simulink model "cantx_0x191"  (R2015a)
settings: Solver=ode45  SolverMode=SingleTasking  StartTime=0.0  StopTime=10.0  RelTol=1e-3
libraries: simulink x6
settings Model: CovMetricSettings=dwe  CovHtmlReporting=off  covSaveCumulativeToWorkspaceVar=off  CovSaveSingleToWorkspaceVar=off  CovExternalEMLEnable=on  Creator=Castiel  LastModifiedBy=Castiel
settings DataIOCC: LimitDataPoints=off  SaveFormat=Dataset  ReturnWorkspaceOutputs=on
settings DebuggingCC: UnconnectedInputMsg=none  UnconnectedOutputMsg=none  UnconnectedLineMsg=none  SFUnexpectedBacktrackingDiag=error  SFNoUnconditionalDefaultTransitionDiag=error
settings HardwareCC: ProdBitPerPointer=64  ProdLargestAtomicFloat=Float  ProdIntDivRoundTo=Zero  ProdEndianess=LittleEndian  ProdHWDeviceType=Specified
settings ModelReferenceCC: PropagateSignalLabelsOutOfModel=on
settings SFSimCC: SimUseLocalCustomCode=on
settings RTWCC: RTWUseLocalCustomCode=on
settings GRTTargetCC: TargetLangStandard=C99 (ISO)

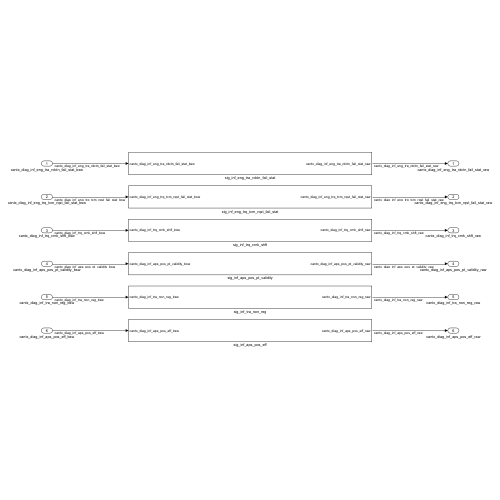
[thumbnail: Simulink's stored preview of the top-level diagram]
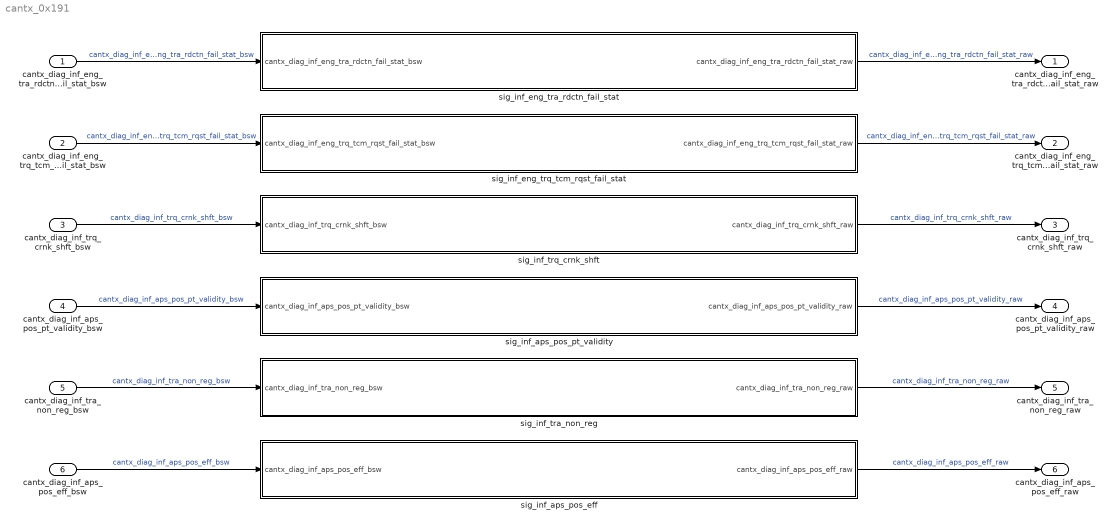
== system cantx_0x191 ==
  cantx_diag_inf_eng_tra_rdctn_fail_stat_bsw : Inport
  cantx_diag_inf_eng_trq_tcm_rqst_fail_stat_bsw : Inport  Port=2
  cantx_diag_inf_trq_crnk_shft_bsw : Inport  Port=3
  cantx_diag_inf_aps_pos_pt_validity_bsw : Inport  Port=4
  cantx_diag_inf_tra_non_reg_bsw : Inport  Port=5
  cantx_diag_inf_aps_pos_eff_bsw : Inport  Port=6
  sig_inf_aps_pos_eff : Subsystem
  sig_inf_aps_pos_pt_validity : Subsystem
  sig_inf_eng_tra_rdctn_fail_stat : Subsystem
  sig_inf_eng_trq_tcm_rqst_fail_stat : Subsystem
  sig_inf_tra_non_reg : Subsystem
  sig_inf_trq_crnk_shft : Subsystem
  cantx_diag_inf_eng_tra_rdctn_fail_stat_raw : Outport
  cantx_diag_inf_eng_trq_tcm_rqst_fail_stat_raw : Outport  Port=2
  cantx_diag_inf_trq_crnk_shft_raw : Outport  Port=3
  cantx_diag_inf_aps_pos_pt_validity_raw : Outport  Port=4
  cantx_diag_inf_tra_non_reg_raw : Outport  Port=5
  cantx_diag_inf_aps_pos_eff_raw : Outport  Port=6
  wires:
  cantx_diag_inf_eng_tra_rdctn_fail_stat_bsw/1 -> sig_inf_eng_tra_rdctn_fail_stat/1(cantx_diag_inf_eng_tra_rdctn_fail_stat_bsw)  "cantx_diag_inf_eng_tra_rdctn_fail_stat_bsw"
  sig_inf_eng_tra_rdctn_fail_stat/1(cantx_diag_inf_eng_tra_rdctn_fail_stat_raw) -> cantx_diag_inf_eng_tra_rdctn_fail_stat_raw/1  "cantx_diag_inf_eng_tra_rdctn_fail_stat_raw"
  cantx_diag_inf_eng_trq_tcm_rqst_fail_stat_bsw/1 -> sig_inf_eng_trq_tcm_rqst_fail_stat/1(cantx_diag_inf_eng_trq_tcm_rqst_fail_stat_bsw)  "cantx_diag_inf_eng_trq_tcm_rqst_fail_stat_bsw"
  sig_inf_eng_trq_tcm_rqst_fail_stat/1(cantx_diag_inf_eng_trq_tcm_rqst_fail_stat_raw) -> cantx_diag_inf_eng_trq_tcm_rqst_fail_stat_raw/1  "cantx_diag_inf_eng_trq_tcm_rqst_fail_stat_raw"
  cantx_diag_inf_trq_crnk_shft_bsw/1 -> sig_inf_trq_crnk_shft/1(cantx_diag_inf_trq_crnk_shft_bsw)  "cantx_diag_inf_trq_crnk_shft_bsw"
  sig_inf_trq_crnk_shft/1(cantx_diag_inf_trq_crnk_shft_raw) -> cantx_diag_inf_trq_crnk_shft_raw/1  "cantx_diag_inf_trq_crnk_shft_raw"
  cantx_diag_inf_aps_pos_pt_validity_bsw/1 -> sig_inf_aps_pos_pt_validity/1(cantx_diag_inf_aps_pos_pt_validity_bsw)  "cantx_diag_inf_aps_pos_pt_validity_bsw"
  sig_inf_aps_pos_pt_validity/1(cantx_diag_inf_aps_pos_pt_validity_raw) -> cantx_diag_inf_aps_pos_pt_validity_raw/1  "cantx_diag_inf_aps_pos_pt_validity_raw"
  cantx_diag_inf_tra_non_reg_bsw/1 -> sig_inf_tra_non_reg/1(cantx_diag_inf_tra_non_reg_bsw)  "cantx_diag_inf_tra_non_reg_bsw"
  sig_inf_tra_non_reg/1(cantx_diag_inf_tra_non_reg_raw) -> cantx_diag_inf_tra_non_reg_raw/1  "cantx_diag_inf_tra_non_reg_raw"
  cantx_diag_inf_aps_pos_eff_bsw/1 -> sig_inf_aps_pos_eff/1(cantx_diag_inf_aps_pos_eff_bsw)  "cantx_diag_inf_aps_pos_eff_bsw"
  sig_inf_aps_pos_eff/1(cantx_diag_inf_aps_pos_eff_raw) -> cantx_diag_inf_aps_pos_eff_raw/1  "cantx_diag_inf_aps_pos_eff_raw"

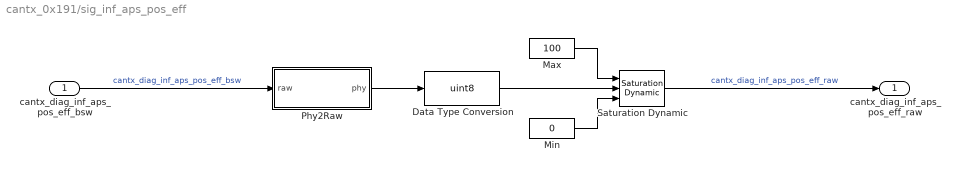
== system cantx_0x191/sig_inf_aps_pos_eff ==
  cantx_diag_inf_aps_pos_eff_bsw : Inport
  Data Type Conversion : DataTypeConversion  OutDataTypeStr=uint8
  Max : Constant  Value=100
  Min : Constant  Value=0
  Phy2Raw : Subsystem  mask{Offset=0, Factor=100/255}
      mask Callback Offset:
      | offset = get_param(gcb, 'Offset');
      |     set_param([gcb, '/Offset'], 'Value', offset);
      mask Callback Factor:
      | factor = get_param(gcb, 'Factor');
      |     set_param([gcb, '/Factor'], 'Value', factor);
      mask Display:
      | disp(['Offset = ', get_param(gcb, 'Offset'), '\n\n']);
      | disp(['Factor = ', get_param(gcb, 'Factor')]);
  Saturation Dynamic : simulink/Discontinuities/Saturation Dynamic  OutMin=[]  OutMax=[]  OutDataTypeStr=Inherit: Same as second input  OutDataType=fixdt(1, 16)  OutScaling=2^-10  DoSatur=off
  cantx_diag_inf_aps_pos_eff_raw : Outport
  wires:
  Saturation Dynamic/1 -> cantx_diag_inf_aps_pos_eff_raw/1  "cantx_diag_inf_aps_pos_eff_raw"
  Phy2Raw/1(phy) -> Data Type Conversion/1
  Data Type Conversion/1 -> Saturation Dynamic/2
  cantx_diag_inf_aps_pos_eff_bsw/1 -> Phy2Raw/1(raw)  "cantx_diag_inf_aps_pos_eff_bsw"
  Min/1 -> Saturation Dynamic/3
  Max/1 -> Saturation Dynamic/1

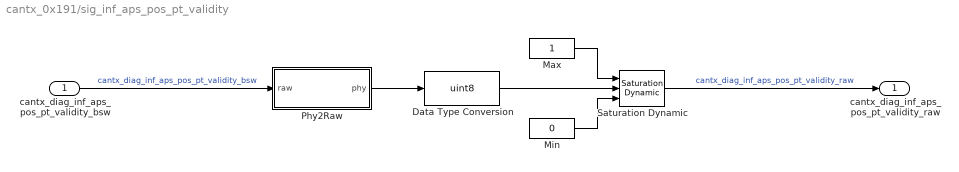
== system cantx_0x191/sig_inf_aps_pos_pt_validity ==
  cantx_diag_inf_aps_pos_pt_validity_bsw : Inport
  Data Type Conversion : DataTypeConversion  OutDataTypeStr=uint8
  Max : Constant
  Min : Constant  Value=0
  Phy2Raw : Subsystem  mask{Offset=0, Factor=1}
      mask Callback Offset:
      | offset = get_param(gcb, 'Offset');
      |     set_param([gcb, '/Offset'], 'Value', offset);
      mask Callback Factor:
      | factor = get_param(gcb, 'Factor');
      |     set_param([gcb, '/Factor'], 'Value', factor);
      mask Display:
      | disp(['Offset = ', get_param(gcb, 'Offset'), '\n\n']);
      | disp(['Factor = ', get_param(gcb, 'Factor')]);
  Saturation Dynamic : simulink/Discontinuities/Saturation Dynamic  OutMin=[]  OutMax=[]  OutDataTypeStr=Inherit: Same as second input  OutDataType=fixdt(1, 16)  OutScaling=2^-10  DoSatur=off
  cantx_diag_inf_aps_pos_pt_validity_raw : Outport
  wires:
  Saturation Dynamic/1 -> cantx_diag_inf_aps_pos_pt_validity_raw/1  "cantx_diag_inf_aps_pos_pt_validity_raw"
  Phy2Raw/1(phy) -> Data Type Conversion/1
  Data Type Conversion/1 -> Saturation Dynamic/2
  cantx_diag_inf_aps_pos_pt_validity_bsw/1 -> Phy2Raw/1(raw)  "cantx_diag_inf_aps_pos_pt_validity_bsw"
  Min/1 -> Saturation Dynamic/3
  Max/1 -> Saturation Dynamic/1

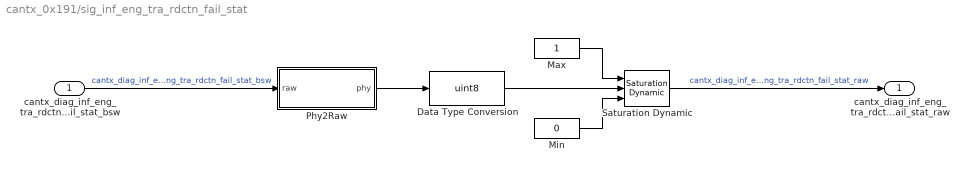
== system cantx_0x191/sig_inf_eng_tra_rdctn_fail_stat ==
  cantx_diag_inf_eng_tra_rdctn_fail_stat_bsw : Inport
  Data Type Conversion : DataTypeConversion  OutDataTypeStr=uint8
  Max : Constant
  Min : Constant  Value=0
  Phy2Raw : Subsystem  mask{Offset=0, Factor=1}
      mask Callback Offset:
      | offset = get_param(gcb, 'Offset');
      |     set_param([gcb, '/Offset'], 'Value', offset);
      mask Callback Factor:
      | factor = get_param(gcb, 'Factor');
      |     set_param([gcb, '/Factor'], 'Value', factor);
      mask Display:
      | disp(['Offset = ', get_param(gcb, 'Offset'), '\n\n']);
      | disp(['Factor = ', get_param(gcb, 'Factor')]);
  Saturation Dynamic : simulink/Discontinuities/Saturation Dynamic  OutMin=[]  OutMax=[]  OutDataTypeStr=Inherit: Same as second input  OutDataType=fixdt(1, 16)  OutScaling=2^-10  DoSatur=off
  cantx_diag_inf_eng_tra_rdctn_fail_stat_raw : Outport
  wires:
  Saturation Dynamic/1 -> cantx_diag_inf_eng_tra_rdctn_fail_stat_raw/1  "cantx_diag_inf_eng_tra_rdctn_fail_stat_raw"
  Phy2Raw/1(phy) -> Data Type Conversion/1
  Data Type Conversion/1 -> Saturation Dynamic/2
  cantx_diag_inf_eng_tra_rdctn_fail_stat_bsw/1 -> Phy2Raw/1(raw)  "cantx_diag_inf_eng_tra_rdctn_fail_stat_bsw"
  Min/1 -> Saturation Dynamic/3
  Max/1 -> Saturation Dynamic/1

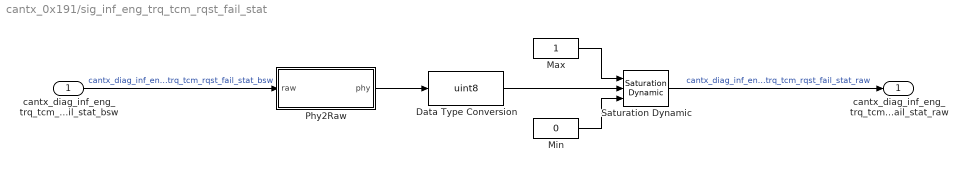
== system cantx_0x191/sig_inf_eng_trq_tcm_rqst_fail_stat ==
  cantx_diag_inf_eng_trq_tcm_rqst_fail_stat_bsw : Inport
  Data Type Conversion : DataTypeConversion  OutDataTypeStr=uint8
  Max : Constant
  Min : Constant  Value=0
  Phy2Raw : Subsystem  mask{Offset=0, Factor=1}
      mask Callback Offset:
      | offset = get_param(gcb, 'Offset');
      |     set_param([gcb, '/Offset'], 'Value', offset);
      mask Callback Factor:
      | factor = get_param(gcb, 'Factor');
      |     set_param([gcb, '/Factor'], 'Value', factor);
      mask Display:
      | disp(['Offset = ', get_param(gcb, 'Offset'), '\n\n']);
      | disp(['Factor = ', get_param(gcb, 'Factor')]);
  Saturation Dynamic : simulink/Discontinuities/Saturation Dynamic  OutMin=[]  OutMax=[]  OutDataTypeStr=Inherit: Same as second input  OutDataType=fixdt(1, 16)  OutScaling=2^-10  DoSatur=off
  cantx_diag_inf_eng_trq_tcm_rqst_fail_stat_raw : Outport
  wires:
  Saturation Dynamic/1 -> cantx_diag_inf_eng_trq_tcm_rqst_fail_stat_raw/1  "cantx_diag_inf_eng_trq_tcm_rqst_fail_stat_raw"
  Phy2Raw/1(phy) -> Data Type Conversion/1
  Data Type Conversion/1 -> Saturation Dynamic/2
  cantx_diag_inf_eng_trq_tcm_rqst_fail_stat_bsw/1 -> Phy2Raw/1(raw)  "cantx_diag_inf_eng_trq_tcm_rqst_fail_stat_bsw"
  Min/1 -> Saturation Dynamic/3
  Max/1 -> Saturation Dynamic/1

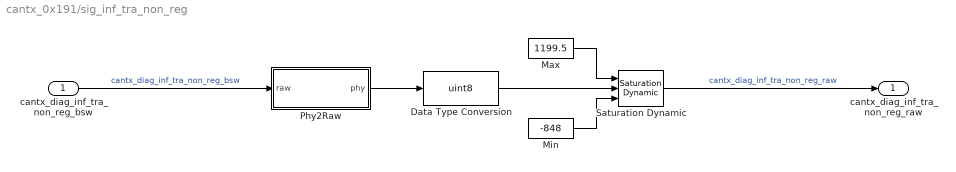
== system cantx_0x191/sig_inf_tra_non_reg ==
  cantx_diag_inf_tra_non_reg_bsw : Inport
  Data Type Conversion : DataTypeConversion  OutDataTypeStr=uint8
  Max : Constant  Value=1199.5
  Min : Constant  Value=-848
  Phy2Raw : Subsystem  mask{Offset=-848, Factor=0.5}
      mask Callback Offset:
      | offset = get_param(gcb, 'Offset');
      |     set_param([gcb, '/Offset'], 'Value', offset);
      mask Callback Factor:
      | factor = get_param(gcb, 'Factor');
      |     set_param([gcb, '/Factor'], 'Value', factor);
      mask Display:
      | disp(['Offset = ', get_param(gcb, 'Offset'), '\n\n']);
      | disp(['Factor = ', get_param(gcb, 'Factor')]);
  Saturation Dynamic : simulink/Discontinuities/Saturation Dynamic  OutMin=[]  OutMax=[]  OutDataTypeStr=Inherit: Same as second input  OutDataType=fixdt(1, 16)  OutScaling=2^-10  DoSatur=off
  cantx_diag_inf_tra_non_reg_raw : Outport
  wires:
  Saturation Dynamic/1 -> cantx_diag_inf_tra_non_reg_raw/1  "cantx_diag_inf_tra_non_reg_raw"
  Phy2Raw/1(phy) -> Data Type Conversion/1
  Data Type Conversion/1 -> Saturation Dynamic/2
  cantx_diag_inf_tra_non_reg_bsw/1 -> Phy2Raw/1(raw)  "cantx_diag_inf_tra_non_reg_bsw"
  Min/1 -> Saturation Dynamic/3
  Max/1 -> Saturation Dynamic/1

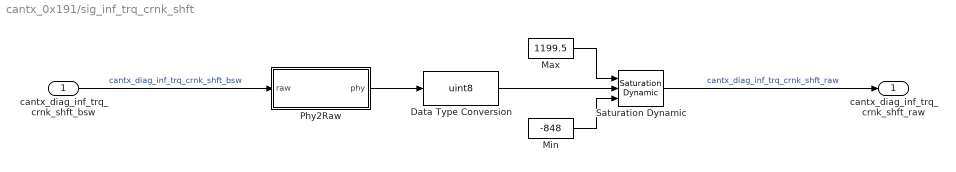
== system cantx_0x191/sig_inf_trq_crnk_shft ==
  cantx_diag_inf_trq_crnk_shft_bsw : Inport
  Data Type Conversion : DataTypeConversion  OutDataTypeStr=uint8
  Max : Constant  Value=1199.5
  Min : Constant  Value=-848
  Phy2Raw : Subsystem  mask{Offset=-848, Factor=0.5}
      mask Callback Offset:
      | offset = get_param(gcb, 'Offset');
      |     set_param([gcb, '/Offset'], 'Value', offset);
      mask Callback Factor:
      | factor = get_param(gcb, 'Factor');
      |     set_param([gcb, '/Factor'], 'Value', factor);
      mask Display:
      | disp(['Offset = ', get_param(gcb, 'Offset'), '\n\n']);
      | disp(['Factor = ', get_param(gcb, 'Factor')]);
  Saturation Dynamic : simulink/Discontinuities/Saturation Dynamic  OutMin=[]  OutMax=[]  OutDataTypeStr=Inherit: Same as second input  OutDataType=fixdt(1, 16)  OutScaling=2^-10  DoSatur=off
  cantx_diag_inf_trq_crnk_shft_raw : Outport
  wires:
  Saturation Dynamic/1 -> cantx_diag_inf_trq_crnk_shft_raw/1  "cantx_diag_inf_trq_crnk_shft_raw"
  Phy2Raw/1(phy) -> Data Type Conversion/1
  Data Type Conversion/1 -> Saturation Dynamic/2
  cantx_diag_inf_trq_crnk_shft_bsw/1 -> Phy2Raw/1(raw)  "cantx_diag_inf_trq_crnk_shft_bsw"
  Min/1 -> Saturation Dynamic/3
  Max/1 -> Saturation Dynamic/1

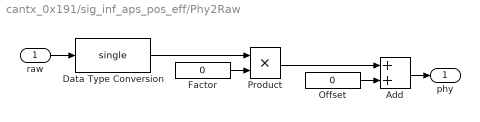
== system cantx_0x191/sig_inf_aps_pos_eff/Phy2Raw ==
  raw : Inport
  Add : Sum
  Data Type Conversion : DataTypeConversion  OutDataTypeStr=single
  Factor : Constant  Value=0
  Offset : Constant  Value=0
  Product : Product
  phy : Outport
  wires:
  Add/1 -> phy/1
  Factor/1 -> Product/2
  Data Type Conversion/1 -> Product/1
  Offset/1 -> Add/2
  Product/1 -> Add/1
  raw/1 -> Data Type Conversion/1

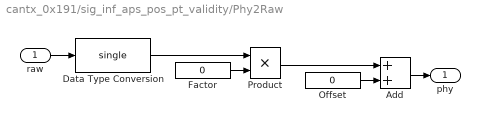
== system cantx_0x191/sig_inf_aps_pos_pt_validity/Phy2Raw ==
  raw : Inport
  Add : Sum
  Data Type Conversion : DataTypeConversion  OutDataTypeStr=single
  Factor : Constant  Value=0
  Offset : Constant  Value=0
  Product : Product
  phy : Outport
  wires:
  Add/1 -> phy/1
  Factor/1 -> Product/2
  Data Type Conversion/1 -> Product/1
  Offset/1 -> Add/2
  Product/1 -> Add/1
  raw/1 -> Data Type Conversion/1

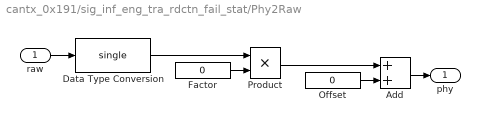
== system cantx_0x191/sig_inf_eng_tra_rdctn_fail_stat/Phy2Raw ==
  raw : Inport
  Add : Sum
  Data Type Conversion : DataTypeConversion  OutDataTypeStr=single
  Factor : Constant  Value=0
  Offset : Constant  Value=0
  Product : Product
  phy : Outport
  wires:
  Add/1 -> phy/1
  Factor/1 -> Product/2
  Data Type Conversion/1 -> Product/1
  Offset/1 -> Add/2
  Product/1 -> Add/1
  raw/1 -> Data Type Conversion/1

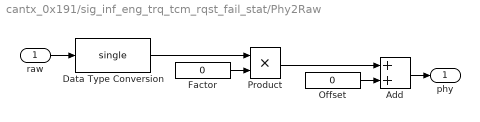
== system cantx_0x191/sig_inf_eng_trq_tcm_rqst_fail_stat/Phy2Raw ==
  raw : Inport
  Add : Sum
  Data Type Conversion : DataTypeConversion  OutDataTypeStr=single
  Factor : Constant  Value=0
  Offset : Constant  Value=0
  Product : Product
  phy : Outport
  wires:
  Add/1 -> phy/1
  Factor/1 -> Product/2
  Data Type Conversion/1 -> Product/1
  Offset/1 -> Add/2
  Product/1 -> Add/1
  raw/1 -> Data Type Conversion/1

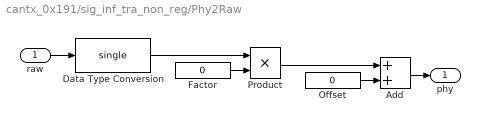
== system cantx_0x191/sig_inf_tra_non_reg/Phy2Raw ==
  raw : Inport
  Add : Sum
  Data Type Conversion : DataTypeConversion  OutDataTypeStr=single
  Factor : Constant  Value=0
  Offset : Constant  Value=0
  Product : Product
  phy : Outport
  wires:
  Add/1 -> phy/1
  Factor/1 -> Product/2
  Data Type Conversion/1 -> Product/1
  Offset/1 -> Add/2
  Product/1 -> Add/1
  raw/1 -> Data Type Conversion/1

== system cantx_0x191/sig_inf_trq_crnk_shft/Phy2Raw ==
  raw : Inport
  Add : Sum
  Data Type Conversion : DataTypeConversion  OutDataTypeStr=single
  Factor : Constant  Value=0
  Offset : Constant  Value=0
  Product : Product
  phy : Outport
  wires:
  Add/1 -> phy/1
  Factor/1 -> Product/2
  Data Type Conversion/1 -> Product/1
  Offset/1 -> Add/2
  Product/1 -> Add/1
  raw/1 -> Data Type Conversion/1
